simulink model "demod_my_cpm"  (R2014b)
settings: Solver=ode45  StartTime=0.0  StopTime=0.12  RelTol=1e-3
libraries: commsink2 x4, siglabs_lib x3, commdigbbndcpm2 x1
settings Model: NumberOfSteps=100  Creator=Ben  LastModifiedBy=Ben

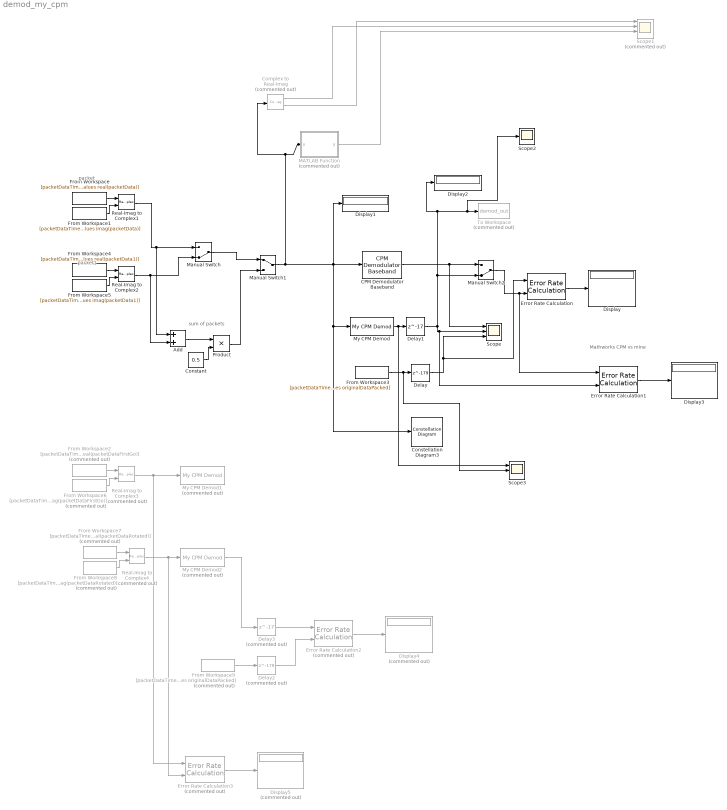
== system demod_my_cpm ==
  note: Mathworks CPM vs mine
  note: sum of packets
  note: packet1
  note: packet
  Add : Sum
  CPM Demodulator Baseband : commdigbbndcpm2/CPM Demodulator Baseband  Mnum=2  outputType=Integer  mappingType=Binary  modIdx=2  pulseShape=Rectangular  BT=0.3  mainLobePulseLength=1  rollOff=0.2  pulseLength=1  preHistory=1  phaseOffset=0  samplesPerSymbol=10  RateOptions=Allow multirate processing  traceBack=16  outDType=double
  Complex to Real-Imag : ComplexToRealImag  Commented=on
  Constant : Constant  Value=0.5
  Constellation Diagram3 : ConstellationDiagram
  Delay : Delay  DelayLength=179  InitialCondition=0
  Delay1 : Delay  DelayLength=17  InitialCondition=0
  Delay2 : Delay  Commented=on  DelayLength=179  InitialCondition=0
  Delay3 : Delay  Commented=on  DelayLength=17  InitialCondition=0
  Display{,1..3} (4 alike) : Display
  Display4 : Display  Commented=on
  Display5 : Display  Commented=on
  Error Rate Calculation : commsink2/Error Rate Calculation  N=0  st_delay=180  cp_mode=Entire frame  subframe=[]  PMode=Port  WsName=ErrorVec  RsMode2=off  stop=off  numErr=100  maxBits=1e6
  Error Rate Calculation1 : commsink2/Error Rate Calculation  N=0  st_delay=180  cp_mode=Entire frame  subframe=[]  PMode=Port  WsName=ErrorVec  RsMode2=off  stop=off  numErr=100  maxBits=1e6
  Error Rate Calculation2 : commsink2/Error Rate Calculation  Commented=on  N=0  st_delay=180  cp_mode=Entire frame  subframe=[]  PMode=Port  WsName=ErrorVec  RsMode2=off  stop=off  numErr=100  maxBits=1e6
  Error Rate Calculation3 : commsink2/Error Rate Calculation  Commented=on  N=0  st_delay=180  cp_mode=Entire frame  subframe=[]  PMode=Port  WsName=ErrorVec  RsMode2=off  stop=off  numErr=100  maxBits=1e6
  From Workspace : FromWorkspace  VariableName=[packetDataTimeValues real(packetData)]  OutDataTypeStr=double  SampleTime=1/(10000*10)  Interpolate=off  OutputAfterFinalValue=Setting to zero
  From Workspace1 : FromWorkspace  VariableName=[packetDataTimeValues imag(packetData)]  OutDataTypeStr=double  SampleTime=1/(10000*10)  Interpolate=off  OutputAfterFinalValue=Setting to zero
  From Workspace2 : FromWorkspace  Commented=on  VariableName=[packetDataTimeValues real(packetDataFirstGo)]  OutDataTypeStr=double  SampleTime=1/(10000*10)  Interpolate=off  OutputAfterFinalValue=Setting to zero
  From Workspace3 : FromWorkspace  VariableName=[packetDataTimeValues originalDataPacked]  OutDataTypeStr=double  SampleTime=1/(10000*10)  Interpolate=off  OutputAfterFinalValue=Setting to zero
  From Workspace4 : FromWorkspace  VariableName=[packetDataTimeValues real(packetData1)]  OutDataTypeStr=double  SampleTime=1/(10000*10)  Interpolate=off  OutputAfterFinalValue=Setting to zero
  From Workspace5 : FromWorkspace  VariableName=[packetDataTimeValues imag(packetData1)]  OutDataTypeStr=double  SampleTime=1/(10000*10)  Interpolate=off  OutputAfterFinalValue=Setting to zero
  From Workspace6 : FromWorkspace  Commented=on  VariableName=[packetDataTimeValues imag(packetDataFirstGo)]  OutDataTypeStr=double  SampleTime=1/(10000*10)  Interpolate=off  OutputAfterFinalValue=Setting to zero
  From Workspace7 : FromWorkspace  Commented=on  VariableName=[packetDataTimeValues real(packetDataRotated)]  OutDataTypeStr=double  SampleTime=1/(10000*10)  Interpolate=off  OutputAfterFinalValue=Setting to zero
  From Workspace8 : FromWorkspace  Commented=on  VariableName=[packetDataTimeValues imag(packetDataRotated)]  OutDataTypeStr=double  SampleTime=1/(10000*10)  Interpolate=off  OutputAfterFinalValue=Setting to zero
  From Workspace9 : FromWorkspace  Commented=on  VariableName=[packetDataTimeValues originalDataPacked]  OutDataTypeStr=double  SampleTime=1/(10000*10)  Interpolate=off  OutputAfterFinalValue=Setting to zero
  MATLAB Function : MATLAB Function  Commented=on  TreatAsAtomicUnit=on
  Manual Switch : ManualSwitch  CurrentSetting=0
  Manual Switch1 : ManualSwitch
  Manual Switch2 : ManualSwitch  CurrentSetting=0
  My CPM Demod : siglabs_lib/My CPM Demod  SampsPerSym=10  RotationsPerSym=1
  My CPM Demod1 : siglabs_lib/My CPM Demod  Commented=on  SampsPerSym=10  RotationsPerSym=1
  My CPM Demod2 : siglabs_lib/My CPM Demod  Commented=on  SampsPerSym=10  RotationsPerSym=1
  Product : Product
  Real-Imag to Complex1 : RealImagToComplex
  Real-Imag to Complex2 : RealImagToComplex
  Real-Imag to Complex3 : RealImagToComplex  Commented=on
  Real-Imag to Complex4 : RealImagToComplex  Commented=on
  Scope : Scope  NumInputPorts=3
      settings: TimeRange=0.01  YMin=-1~-1~-1  YMax=1~1~1
  Scope1 : Scope  Commented=on  NumInputPorts=4
      settings: TimeRange=0.001  YMin=-1~-1~-5~-5  YMax=1~1~5~5
  Scope2 : Scope
      settings: TimeRange=0.01  YMin=-1  YMax=1  SaveName=ScopeData2
  Scope3 : Scope  NumInputPorts=3
      settings: TimeRange=0.01  YMin=-1~-1~-1  YMax=1~1~1  SaveName=ScopeData3
  To Workspace : ToWorkspace  Commented=on  VariableName=demod_out  SampleTime=-1
  wires:
  From Workspace1/1 -> Real-Imag to Complex1/2
  From Workspace/1 -> Real-Imag to Complex1/1
  Real-Imag to Complex1/1 -> Add/1, Manual Switch/1
  From Workspace3/1 -> Scope3/2, Delay/1
  Delay/1 -> Error Rate Calculation/1, Scope/3
  CPM Demodulator Baseband/1 -> Manual Switch2/1, Scope/1
  From Workspace5/1 -> Real-Imag to Complex2/2
  From Workspace4/1 -> Real-Imag to Complex2/1
  Manual Switch/1 -> Manual Switch1/1
  Real-Imag to Complex2/1 -> Add/2, Manual Switch/2
  Error Rate Calculation/1 -> Display/1
  Add/1 -> Product/1
  Constant/1 -> Product/2
  Manual Switch1/1 -> Display1/1, Constellation Diagram3/1, My CPM Demod/1, CPM Demodulator Baseband/1, MATLAB Function/1(u), Complex to Real-Imag/1
  Product/1 -> Manual Switch1/2
  My CPM Demod/1 -> Scope3/1, Delay1/1
  Complex to Real-Imag/2 -> Scope1/1
  Complex to Real-Imag/1 -> Scope1/2
  MATLAB Function/1(y) -> Scope1/3
  Delay1/1 -> Error Rate Calculation1/2, Scope/2, Manual Switch2/2, Display2/1, Scope2/1, To Workspace/1
  Error Rate Calculation1/1 -> Display3/1
  Manual Switch2/1 -> Error Rate Calculation1/1, Error Rate Calculation/2
  From Workspace6/1 -> Real-Imag to Complex3/2
  From Workspace2/1 -> Real-Imag to Complex3/1
  From Workspace8/1 -> Real-Imag to Complex4/2
  From Workspace7/1 -> Real-Imag to Complex4/1
  Real-Imag to Complex3/1 -> Error Rate Calculation3/1, My CPM Demod1/1
  Real-Imag to Complex4/1 -> Error Rate Calculation3/2, My CPM Demod2/1
  Error Rate Calculation2/1 -> Display4/1
  From Workspace9/1 -> Delay2/1
  Delay3/1 -> Error Rate Calculation2/1
  Delay2/1 -> Error Rate Calculation2/2
  My CPM Demod2/1 -> Delay3/1
  Error Rate Calculation3/1 -> Display5/1

== matlab function demod_my_cpm/MATLAB Function ==
  data: u input; y output
function y = fcn(u)
%#codegen

y = angle(u);
